simulink model "emrax208"  (R2024a)
settings: Solver=ode5  StartTime=0.0  StopTime=sim.time  FixedStep=sim.Ts  RelTol=1e-3
undefined symbols (not defined in the file or in its folder): c, ki, kp, sim, T_ref
libraries: slpidlib x2, simulink x1
settings Model: SimulationMode=accelerator  Creator=skh88  LastModifiedBy=skh88
settings SimscapeCC: ExplicitSolverDiagnosticOptions=none

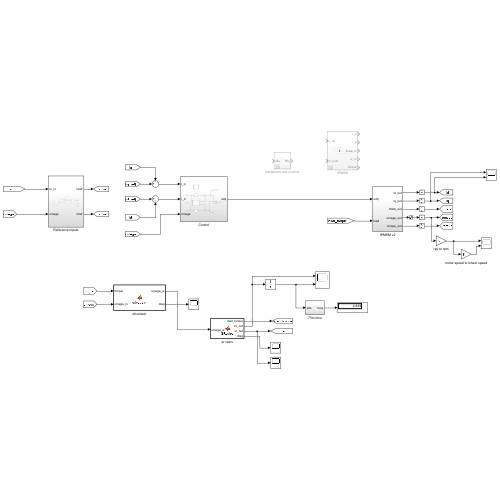
[thumbnail: Simulink's stored preview of the top-level diagram]
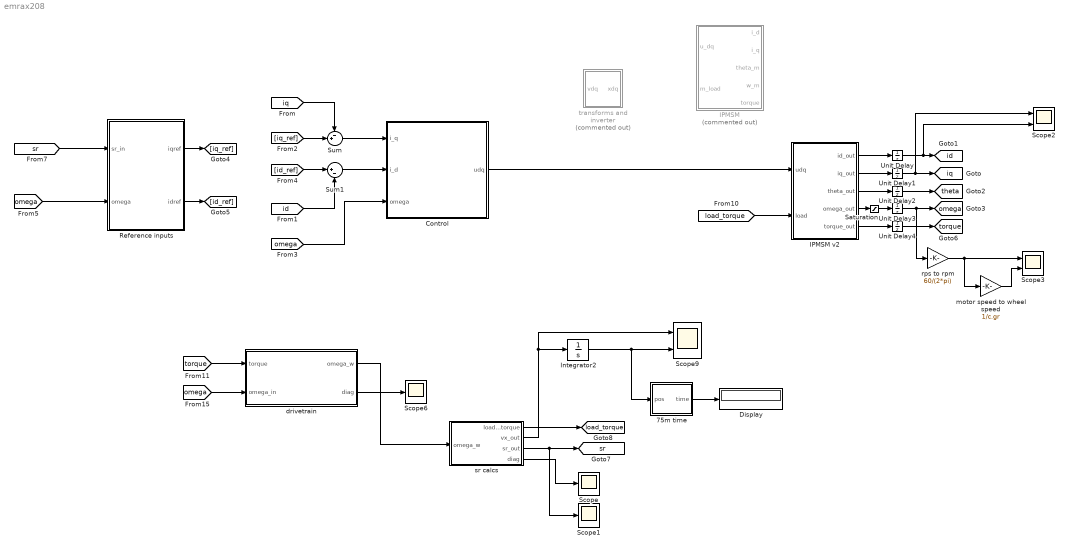
== system emrax208 ==
  75m time : Subsystem
  Control : Subsystem
  Display : Display
  IPMSM : Subsystem  Commented=on
  IPMSM v2 : Subsystem
  Integrator2 : Integrator
  Reference inputs : Subsystem
  Saturation : Saturate  UpperLimit=c.max_rpm  LowerLimit=0
  Scope : Scope
  Scope1 : Scope
  Scope2 : Scope  NumInputPorts=2
  Scope3 : Scope  NumInputPorts=2
  Scope6 : Scope
  Scope9 : Scope  NumInputPorts=2
  Sum : Sum  Inputs=-+|
  Sum1 : Sum  Inputs=|+-
  Unit Delay{,1..4} (5 alike) : UnitDelay  SampleTime=-1  HasFrameUpgradeWarning=on
  drivetrain : MATLAB Function  TreatAsAtomicUnit=on
  motor speed to wheel speed : Gain  Gain=1/c.gr
  rps to rpm : Gain  Gain=60/(2*pi)
  sr calcs : MATLAB Function  TreatAsAtomicUnit=on
  transforms and inverter : Subsystem  Commented=on
  tag scope: id=global, iq=global, load_torque=global, omega=global, sr=global, theta=global, torque=global
  wires:
  [iq] -> Sum/1
  [id] -> Sum1/2
  Reference inputs/1(iqref) -> [iq_ref]
  Reference inputs/2(idref) -> [id_ref]
  [iq_ref] -> Sum/2
  [id_ref] -> Sum1/1
  rps to rpm/1 -> Scope3/1, motor speed to wheel speed/1
  motor speed to wheel speed/1 -> Scope3/2
  Sum/1 -> Control/1(i_q)
  Sum1/1 -> Control/2(i_d)
  [omega] -> Control/3(omega)
  Unit Delay/1 -> Scope2/2, [id]
  Unit Delay1/1 -> Scope2/1, [iq]
  Unit Delay4/1 -> [torque]
  Unit Delay2/1 -> [theta]
  Unit Delay3/1 -> [omega], rps to rpm/1
  IPMSM v2/3(theta_out) -> Unit Delay2/1
  IPMSM v2/2(iq_out) -> Unit Delay1/1
  IPMSM v2/1(id_out) -> Unit Delay/1
  IPMSM v2/4(omega_out) -> Saturation/1
  IPMSM v2/5(torque_out) -> Unit Delay4/1
  Saturation/1 -> Unit Delay3/1
  [load_torque] -> IPMSM v2/2(load)
  sr calcs/2(vx_out) -> Integrator2/1, Scope9/1
  drivetrain/2(diag) -> Scope6/1
  Integrator2/1 -> 75m time/1(pos), Scope9/2
  sr calcs/4(diag) -> Scope/1
  drivetrain/1(omega_w) -> sr calcs/1(omega_w)
  75m time/1(time) -> Display/1
  [omega] -> drivetrain/2(omega_in)
  sr calcs/1(load_torque) -> [load_torque]
  sr calcs/3(sr_out) -> Scope1/1, [sr]
  [torque] -> drivetrain/1(torque)
  [sr] -> Reference inputs/1(sr_in)
  [omega] -> Reference inputs/2(omega)
  Control/1(udq) -> IPMSM v2/1(udq)

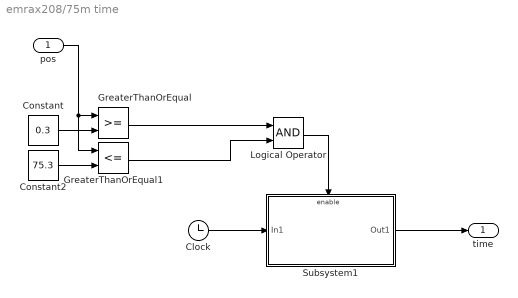
== system emrax208/75m time ==
  pos : Inport
  Clock : Clock
  Constant : Constant  Value=0.3
  Constant2 : Constant  Value=75.3
  GreaterThanOrEqual : RelationalOperator  OutDataTypeStr=boolean  RndMeth=Simplest  InputSameDT=off
  GreaterThanOrEqual1 : RelationalOperator  Operator=<=  OutDataTypeStr=boolean  RndMeth=Simplest  InputSameDT=off
  Logical Operator : Logic  AllPortsSameDT=off  OutDataTypeStr=boolean
  Subsystem1 : Subsystem
  time : Outport
  wires:
  Constant/1 -> GreaterThanOrEqual/2
  Logical Operator/1 -> Subsystem1/Enable
  GreaterThanOrEqual1/1 -> Logical Operator/2
  Clock/1 -> Subsystem1/1(In1)
  Constant2/1 -> GreaterThanOrEqual1/2
  Subsystem1/1(Out1) -> time/1
  GreaterThanOrEqual/1 -> Logical Operator/1
  pos/1 -> GreaterThanOrEqual1/1, GreaterThanOrEqual/1

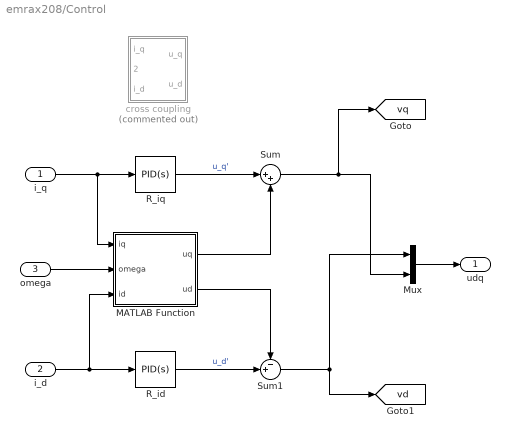
== system emrax208/Control ==
  i_q : Inport
  i_d : Inport  Port=2
  omega : Inport  Port=3
  MATLAB Function : MATLAB Function  TreatAsAtomicUnit=on
  Mux : Mux  Inputs=2
  R_id : slpidlib/PID Controller  Controller=PID  Form=Parallel  TimeDomain=Continuous-time  UseExternalTs=off  SampleTime=c.controllerTs  IntegratorMethod=Forward Euler  FilterMethod=Forward Euler  ControllerParametersSource=internal  P=kp  I=ki  UseKiTs=off  D=0  UseExternalDerivativeSource=off  N=100  UseFilter=on  TunerSelectOption=Transfer Function Based (PID Tuner App)  InitialConditionSource=internal  InitialConditionForIntegrator=0  InitialConditionForFilter=0  DifferentiatorICPrevScaledInput=0  ExternalReset=none  TrackingMode=off  Kt=1  LimitOutput=off  SatLimitsSource=internal  UpperSaturationLimit=2*c.R*c.I_nominal  LowerSaturationLimit=-2*c.R*c.I_nominal  LinearizeAsGain=on  AntiWindupMode=clamping  Kb=1  LimitIntegrator=off  UpperIntegratorSaturationLimit=2*c.R*c.I_nominal  LowerIntegratorSaturationLimit=-2*c.R*c.I_nominal  POutMin=[]  POutMax=[]  IOutMin=[]  IOutMax=[]  DOutMin=[]  DOutMax=[]  NOutMin=[]  NOutMax=[]  SumOutMin=[]  SumOutMax=[]  SaturationOutMin=[]  SaturationOutMax=[]  PParamMin=[]  PParamMax=[]  IParamMin=[]  IParamMax=[]  DParamMin=[]  DParamMax=[]  NParamMin=[]  NParamMax=[]  KbParamMin=[]  KbParamMax=[]  KtParamMin=[]  KtParamMax=[]  KbOutMin=[]  KbOutMax=[]  KtOutMin=[]  KtOutMax=[]  IntegratorOutMin=[]  IntegratorOutMax=[]  FilterOutMin=[]  FilterOutMax=[]  SumI1OutMin=[]  SumI1OutMax=[]  SumI2OutMin=[]  SumI2OutMax=[]  SumI3OutMin=[]  SumI3OutMax=[]  SumI4OutMin=[]  SumI4OutMax=[]  SumDOutMin=[]  SumDOutMax=[]  DifferentiatorOutMin=[]  DifferentiatorOutMax=[]  FilterDiffOutCoefMin=[]  FilterDiffOutCoefMax=[]  ReciprocalOutMin=[]  ReciprocalOutMax=[]  SumDenOutMin=[]  SumDenOutMax=[]  SumNumOutMin=[]  SumNumOutMax=[]  DivideOutMin=[]  DivideOutMax=[]  UdiffTsProdOutMin=[]  UdiffTsProdOutMax=[]  NTsProdOutMin=[]  NTsProdOutMax=[]  UintegralTsProdOutMin=[]  UintegralTsProdOutMax=[]  UngainTsProdOutMin=[]  UngainTsProdOutMax=[]  ClampingZeroOutDataTypeStr=Inherit: Inherit via back propagation  ClampingZeroOutMin=[]  ClampingZeroOutMax=[]  FilterDenConstantOutDataTypeStr=Inherit: Inherit via back propagation  FilterDenConstantOutMin=[]  FilterDenConstantOutMax=[]  PCopyOutDataTypeStr=Inherit: Inherit via back propagation  PCopyOutMin=[]  PCopyOutMax=[]  NCopyOutDataTypeStr=Inherit: Inherit via back propagation  NCopyOutMin=[]  NCopyOutMax=[]  IntegratorContinuousStateAttributes=''  IntegratorStateMustResolveToSignalObject=off  IntegratorRTWStateStorageClass=Auto  FilterContinuousStateAttributes=''  FilterStateMustResolveToSignalObject=off  FilterRTWStateStorageClass=Auto  ParallelPVariant=InternalParameters  IdealPVariant=Disabled  IVariant=InternalParameters  DVariant=InternalParameters  IntegratorVariant=Continuous  SatVariant=Disabled  AWVariant=Passthrough  PCopyVariant=Disabled  TRVariant=Disabled  FdbkBlocksVariant=Forward  IdealPFdbkVariant=Disabled  SatFdbkVariant=Disabled  DerivativeFilterVariant=ContFilter  NVariant=InternalParameters  NCopyVariant=Disabled  FilterICVariant=InternalICsFilter  IntegratorICVariant=InternalICs  ExternalResetVariant=Disabled  TRSumVariant=Passthrough  SumFdbkVariant=Disabled  SumVariant=Sum_PID  TsampFilterVariant=InternalTs  TsampNgainVariant=Passthrough  TsampIntegralVariant=Disabled_SignalSpec  ExternalSaturationOutDataTypeStr=Inherit: Same as second input  DerivativeSourceVariant=ErrorSignal
  R_iq : slpidlib/PID Controller  Controller=PID  Form=Parallel  TimeDomain=Continuous-time  UseExternalTs=off  SampleTime=c.controllerTs  IntegratorMethod=Forward Euler  FilterMethod=Forward Euler  ControllerParametersSource=internal  P=kp  I=ki  UseKiTs=off  D=0  UseExternalDerivativeSource=off  N=100  UseFilter=on  TunerSelectOption=Transfer Function Based (PID Tuner App)  InitialConditionSource=internal  InitialConditionForIntegrator=0  InitialConditionForFilter=0  DifferentiatorICPrevScaledInput=0  ExternalReset=none  TrackingMode=off  Kt=1  LimitOutput=off  SatLimitsSource=internal  UpperSaturationLimit=c.max_rpm*c.p*c.lambda  LowerSaturationLimit=-c.max_rpm*c.p*c.lambda  LinearizeAsGain=on  AntiWindupMode=clamping  Kb=1  LimitIntegrator=off  UpperIntegratorSaturationLimit=c.max_rpm*c.p*c.lambda  LowerIntegratorSaturationLimit=-c.max_rpm*c.p*c.lambda  POutMin=[]  POutMax=[]  IOutMin=[]  IOutMax=[]  DOutMin=[]  DOutMax=[]  NOutMin=[]  NOutMax=[]  SumOutMin=[]  SumOutMax=[]  SaturationOutMin=[]  SaturationOutMax=[]  PParamMin=[]  PParamMax=[]  IParamMin=[]  IParamMax=[]  DParamMin=[]  DParamMax=[]  NParamMin=[]  NParamMax=[]  KbParamMin=[]  KbParamMax=[]  KtParamMin=[]  KtParamMax=[]  KbOutMin=[]  KbOutMax=[]  KtOutMin=[]  KtOutMax=[]  IntegratorOutMin=[]  IntegratorOutMax=[]  FilterOutMin=[]  FilterOutMax=[]  SumI1OutMin=[]  SumI1OutMax=[]  SumI2OutMin=[]  SumI2OutMax=[]  SumI3OutMin=[]  SumI3OutMax=[]  SumI4OutMin=[]  SumI4OutMax=[]  SumDOutMin=[]  SumDOutMax=[]  DifferentiatorOutMin=[]  DifferentiatorOutMax=[]  FilterDiffOutCoefMin=[]  FilterDiffOutCoefMax=[]  ReciprocalOutMin=[]  ReciprocalOutMax=[]  SumDenOutMin=[]  SumDenOutMax=[]  SumNumOutMin=[]  SumNumOutMax=[]  DivideOutMin=[]  DivideOutMax=[]  UdiffTsProdOutMin=[]  UdiffTsProdOutMax=[]  NTsProdOutMin=[]  NTsProdOutMax=[]  UintegralTsProdOutMin=[]  UintegralTsProdOutMax=[]  UngainTsProdOutMin=[]  UngainTsProdOutMax=[]  ClampingZeroOutDataTypeStr=Inherit: Inherit via back propagation  ClampingZeroOutMin=[]  ClampingZeroOutMax=[]  FilterDenConstantOutDataTypeStr=Inherit: Inherit via back propagation  FilterDenConstantOutMin=[]  FilterDenConstantOutMax=[]  PCopyOutDataTypeStr=Inherit: Inherit via back propagation  PCopyOutMin=[]  PCopyOutMax=[]  NCopyOutDataTypeStr=Inherit: Inherit via back propagation  NCopyOutMin=[]  NCopyOutMax=[]  IntegratorContinuousStateAttributes=''  IntegratorStateMustResolveToSignalObject=off  IntegratorRTWStateStorageClass=Auto  FilterContinuousStateAttributes=''  FilterStateMustResolveToSignalObject=off  FilterRTWStateStorageClass=Auto  ParallelPVariant=InternalParameters  IdealPVariant=Disabled  IVariant=InternalParameters  DVariant=InternalParameters  IntegratorVariant=Continuous  SatVariant=Disabled  AWVariant=Passthrough  PCopyVariant=Disabled  TRVariant=Disabled  FdbkBlocksVariant=Forward  IdealPFdbkVariant=Disabled  SatFdbkVariant=Disabled  DerivativeFilterVariant=ContFilter  NVariant=InternalParameters  NCopyVariant=Disabled  FilterICVariant=InternalICsFilter  IntegratorICVariant=InternalICs  ExternalResetVariant=Disabled  TRSumVariant=Passthrough  SumFdbkVariant=Disabled  SumVariant=Sum_PID  TsampFilterVariant=InternalTs  TsampNgainVariant=Passthrough  TsampIntegralVariant=Disabled_SignalSpec  ExternalSaturationOutDataTypeStr=Inherit: Same as second input  DerivativeSourceVariant=ErrorSignal
  Sum : Sum  Inputs=|++
  Sum1 : Sum  Inputs=-+|
  cross coupling : Subsystem  Commented=on
  udq : Outport
  tag scope: vd=global, vq=global
  wires:
  R_id/1 -> Sum1/2  "u_d'"
  R_iq/1 -> Sum/1  "u_q'"
  i_d/1 -> MATLAB Function/3(id), R_id/1
  i_q/1 -> MATLAB Function/1(iq), R_iq/1
  Sum/1 -> [vq], Mux/2
  omega/1 -> MATLAB Function/2(omega)
  MATLAB Function/1(uq) -> Sum/2
  MATLAB Function/2(ud) -> Sum1/1
  Sum1/1 -> [vd], Mux/1
  Mux/1 -> udq/1

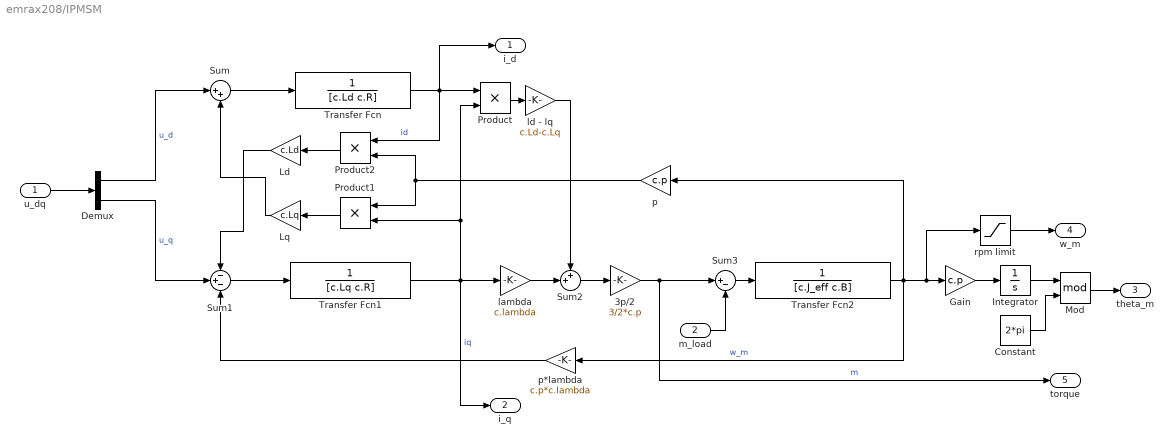
== system emrax208/IPMSM ==
  u_dq : Inport
  m_load : Inport  Port=2
  3p/2 : Gain  Gain=3/2*c.p
  Constant : Constant  Value=2*pi
  Demux : Demux  Outputs=2
  Gain : Gain  Gain=c.p
  Integrator : Integrator
  Ld : Gain  Gain=c.Ld
  Lq : Gain  Gain=c.Lq
  Mod : Math  Operator=mod
  Product : Product
  Product1 : Product
  Product2 : Product
  Sum : Sum  Inputs=|++
  Sum1 : Sum  Inputs=-+-
  Sum2 : Sum  Inputs=++|
  Sum3 : Sum  Inputs=|+-
  Transfer Fcn : TransferFcn  Denominator=[c.Ld c.R]
  Transfer Fcn1 : TransferFcn  Denominator=[c.Lq c.R]
  Transfer Fcn2 : TransferFcn  Denominator=[c.J_eff c.B]
  lambda : Gain  Gain=c.lambda
  ld - lq : Gain  Gain=c.Ld-c.Lq
  p : Gain  Gain=c.p
  p*lambda : Gain  Gain=c.p*c.lambda
  rpm limit : Saturate  UpperLimit=c.max_rpm  LowerLimit=0
  i_d : Outport
  i_q : Outport  Port=2
  theta_m : Outport  Port=3
  w_m : Outport  Port=4
  torque : Outport  Port=5
  wires:
  m_load/1 -> Sum3/2
  Transfer Fcn1/1 -> Product1/2, Product/2, lambda/1, i_q/1  "iq"
  Product2/1 -> Ld/1
  Transfer Fcn/1 -> Product2/1, Product/1, i_d/1  "id"
  p/1 -> Product1/1, Product2/2
  Sum1/1 -> Transfer Fcn1/1
  Sum/1 -> Transfer Fcn/1
  3p/2/1 -> torque/1, Sum3/1  "m"
  Sum3/1 -> Transfer Fcn2/1
  Transfer Fcn2/1 -> p*lambda/1, p/1, Gain/1, rpm limit/1  "w_m"
  lambda/1 -> Sum2/2
  Product1/1 -> Lq/1
  Lq/1 -> Sum/2
  Ld/1 -> Sum1/1
  p*lambda/1 -> Sum1/3
  Integrator/1 -> Mod/1
  rpm limit/1 -> w_m/1
  Demux/1 -> Sum/1  "u_d"
  Demux/2 -> Sum1/2  "u_q"
  u_dq/1 -> Demux/1
  Gain/1 -> Integrator/1
  ld - lq/1 -> Sum2/1
  Sum2/1 -> 3p/2/1
  Product/1 -> ld - lq/1
  Constant/1 -> Mod/2
  Mod/1 -> theta_m/1

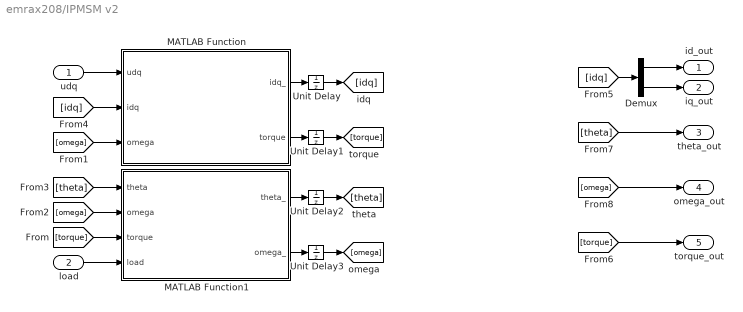
== system emrax208/IPMSM v2 ==
  udq : Inport
  load : Inport  Port=2
  Demux : Demux  Outputs=2
  MATLAB Function : MATLAB Function  TreatAsAtomicUnit=on
  MATLAB Function1 : MATLAB Function  TreatAsAtomicUnit=on
  Unit Delay{,1..3} (4 alike) : UnitDelay  SampleTime=-1  HasFrameUpgradeWarning=on
  id_out : Outport
  iq_out : Outport  Port=2
  theta_out : Outport  Port=3
  omega_out : Outport  Port=4
  torque_out : Outport  Port=5
  wires:
  MATLAB Function/2(torque) -> Unit Delay1/1
  [torque] -> MATLAB Function1/3(torque)
  MATLAB Function1/2(omega_) -> Unit Delay3/1
  [omega] -> MATLAB Function/3(omega)
  [omega] -> MATLAB Function1/2(omega)
  MATLAB Function1/1(theta_) -> Unit Delay2/1
  [theta] -> MATLAB Function1/1(theta)
  load/1 -> MATLAB Function1/4(load)
  udq/1 -> MATLAB Function/1(udq)
  MATLAB Function/1(idq_) -> Unit Delay/1
  [idq] -> MATLAB Function/2(idq)
  [idq] -> Demux/1
  [torque] -> torque_out/1
  [theta] -> theta_out/1
  Demux/1 -> id_out/1
  Demux/2 -> iq_out/1
  Unit Delay/1 -> [idq]
  Unit Delay1/1 -> [torque]
  Unit Delay2/1 -> [theta]
  [omega] -> omega_out/1
  Unit Delay3/1 -> [omega]

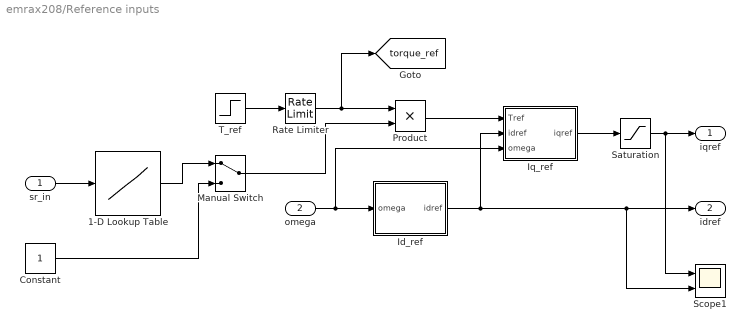
== system emrax208/Reference inputs ==
  sr_in : Inport
  omega : Inport  Port=2
  1-D Lookup Table : Lookup_n-D  NumberOfTableDimensions=1  BreakpointsForDimension1=linspace(0, 0.5, 100)  Table=(-tanh(linspace(-3, 3, 100))+1)/2  InternalRulePriority=Speed  RndMeth=Simplest
  Constant : Constant
  Id_ref : MATLAB Function  TreatAsAtomicUnit=on
  Iq_ref : MATLAB Function  TreatAsAtomicUnit=on
  Manual Switch : ManualSwitch
  Product : Product
  Rate Limiter : RateLimiter  RisingSlewLimit=5e3  FallingSlewLimit=-5e3  SampleTimeMode=inherited
  Saturation : Saturate  UpperLimit=c.I_peak  LowerLimit=-c.I_peak
  Scope1 : Scope  NumInputPorts=2
  T_ref : Step  Time=0  After=T_ref  SampleTime=sim.Ts
  iqref : Outport
  idref : Outport  Port=2
  tag scope: torque_ref=global
  wires:
  Id_ref/1(idref) -> Scope1/2, idref/1, Iq_ref/2(idref)
  Iq_ref/1(iqref) -> Saturation/1
  Saturation/1 -> Scope1/1, iqref/1
  T_ref/1 -> Rate Limiter/1
  Rate Limiter/1 -> [torque_ref], Product/1
  sr_in/1 -> 1-D Lookup Table/1
  Product/1 -> Iq_ref/1(Tref)
  1-D Lookup Table/1 -> Manual Switch/1
  Constant/1 -> Manual Switch/2
  omega/1 -> Iq_ref/3(omega), Id_ref/1(omega)
  Manual Switch/1 -> Product/2

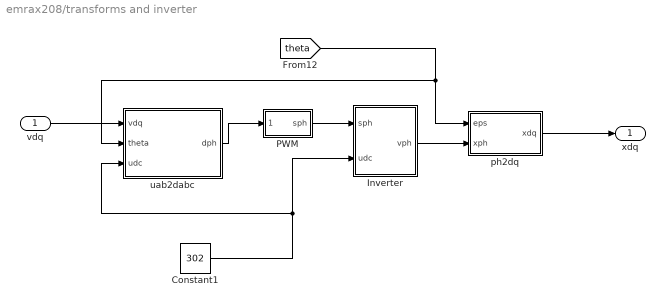
== system emrax208/transforms and inverter ==
  vdq : Inport
  Constant1 : Constant  Value=302  SampleTime=Inf
  Inverter : MATLAB Function  TreatAsAtomicUnit=on
  PWM : Subsystem
  ph2dq : MATLAB Function  TreatAsAtomicUnit=on
  uab2dabc : MATLAB Function  TreatAsAtomicUnit=on
  xdq : Outport
  wires:
  Constant1/1 -> Inverter/2(udc), uab2dabc/3(udc)
  [theta] -> ph2dq/1(eps), uab2dabc/2(theta)
  ph2dq/1(xdq) -> xdq/1
  Inverter/1(vph) -> ph2dq/2(xph)
  uab2dabc/1(dph) -> PWM/1(dph)
  PWM/1(sph) -> Inverter/1(sph)
  vdq/1 -> uab2dabc/1(vdq)

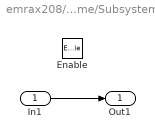
== system emrax208/75m time/Subsystem1 ==
  In1 : Inport
  Enable : EnablePort
  Out1 : Outport
  wires:
  In1/1 -> Out1/1

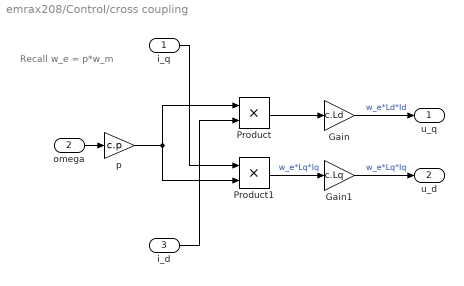
== system emrax208/Control/cross coupling ==
  note: Recall w_e = p*w_m
  i_q : Inport
  omega : Inport  Port=2
  i_d : Inport  Port=3
  Gain : Gain  Gain=c.Ld
  Gain1 : Gain  Gain=c.Lq
  Product : Product
  Product1 : Product
  p : Gain  Gain=c.p
  u_q : Outport
  u_d : Outport  Port=2
  wires:
  i_d/1 -> Product/2
  omega/1 -> p/1
  Gain/1 -> u_q/1  "w_e*Ld*Id"
  i_q/1 -> Product1/1
  Gain1/1 -> u_d/1  "w_e*Lq*Iq"
  p/1 -> Product/1, Product1/2
  Product/1 -> Gain/1
  Product1/1 -> Gain1/1  "w_e*Lq*Iq"

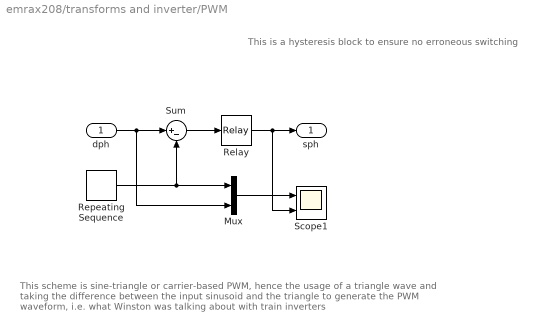
== system emrax208/transforms and inverter/PWM ==
  note: This scheme is sine-triangle or carrier-based PWM, hence the usage of a triangle wave and taking the difference between the input sinusoid and the triangle to generate the PWM waveform, i.e. what Winston was talking about with train inverters
  note: This is a hysteresis block to ensure no erroneous switching
  dph : Inport
  Mux : Mux  Inputs=2
  Relay : Relay  OnSwitchValue=2e-10  OffSwitchValue=-2e-10
  Repeating Sequence : simulink/Sources/Repeating Sequence  rep_seq_t=[0 c.Ts/2 c.Ts]  rep_seq_y=[0 1 0]
  Scope1 : Scope  NumInputPorts=2
  Sum : Sum  Inputs=|+-
  sph : Outport
  wires:
  Sum/1 -> Relay/1
  Repeating Sequence/1 -> Mux/1, Sum/2
  dph/1 -> Mux/2, Sum/1
  Relay/1 -> sph/1, Scope1/2
  Mux/1 -> Scope1/1

== matlab function emrax208/Reference inputs/Id_ref ==
  data: omega input; idref output; c parameter
function idref = fcn(omega, c)

idref = 0;

if omega*c.p >= c.omega_base
    idref = (c.omega_base-omega*c.p)*c.lambda/(omega*c.p*c.Ld);
    idref = max(idref, -c.I_lim);
end

== matlab function emrax208/transforms and inverter/ph2dq ==
  data: eps input; xdq output size=[2,1]; xph input
function xdq  = ph2dq(eps,xph)
  % Synchronous reference frame transformation  
  
  % Space Vector Transformation (Clarke)
  xab=[0;0];
  xab(1)= 2/3*xph(1) - 1/3*(xph(2)+xph(3)); 
  xab(2)= 1/sqrt(3)* (xph(2)-xph(3));
  
  % Direct Vector Calculation (Park)
  xdq=[0;0];
  xdq(1)=  xab(1)*cos(eps) + xab(2)*sin(eps);
  xdq(2)= -xab(1)*sin(eps) + xab(2)*cos(eps);

== matlab function emrax208/IPMSM v2/MATLAB Function ==
  data: idq_ output size=2; torque output size=1; udq input; idq input; omega input; c parameter
function [idq_, torque] = ipmsm_electrical(udq, idq, omega, c)

vd = udq(1) - c.R*idq(1);
vq = udq(2) - c.R*idq(2);

id = (c.Tstep*vd + c.Ld*idq(1) + c.Tstep*omega*c.p*c.Lq*idq(2))/c.Ld;
iq = (c.Tstep*vq + c.Lq*idq(2) - c.Tstep*omega*c.p*(c.Ld*idq(1) + c.lambda))/c.Lq;

idq_ = [id;iq];

torque = 3/2*c.p*(c.lambda*iq + (c.Ld - c.Lq)*id*iq);

== matlab function emrax208/transforms and inverter/uab2dabc ==
  data: dph output size=3; vdq input; theta input; udc input
function dph = fcn(vdq,theta,udc)
%#codegen

% Inverse Park
vab = zeros(2,1);
vab(1) = cos(theta)*vdq(1) -sin(theta)*vdq(2);
vab(2) = sin(theta)*vdq(1) +cos(theta)*vdq(2);

% Inverse Clarke
vph = zeros(3,1);
vph(1) = vab(1);
vph(2) = -1/2*vab(1) +sqrt(3)/2*vab(2);
vph(3) = -1/2*vab(1) -sqrt(3)/2*vab(2);

% modulation index
mph = vph/(udc/2);
% duty cycle
dph = (mph+1)/2;

% limitation
for i=1:3
    if dph(i) > 1
        dph(i) = 1;
    elseif dph(i) < 0
        dph(i) = 0;
    end
end

% backcalculation of applied voltage
vphsat = (2*dph-1)*udc/2;  % m=(2*dph-1)

vabsat = zeros(2,1);
vabsat(1) = 2/3*vphsat(1) -1/3*vphsat(2) -1/3*vphsat(3);
vabsat(2) = 1/sqrt(3)*vphsat(2) -1/sqrt(3)*vphsat(3);

vdqsat = zeros(2,1);
vdqsat(1) =  cos(theta)*vabsat(1) +sin(theta)*vabsat(2);
vdqsat(2) = -sin(theta)*vabsat(1) +cos(theta)*vabsat(2);

== matlab function emrax208/transforms and inverter/Inverter ==
  data: sph input; vph output; udc input
function vph  = fcn(sph,udc)
%#codegen

vph = (2*sph-1)*udc/2;

== matlab function emrax208/IPMSM v2/MATLAB Function1 ==
  data: theta_ output; omega_ output; theta input; omega input; torque input; load input; c parameter
function [theta_, omega_] = ipmsm_mechanical(theta, omega, torque, load, c)

omega_ = c.Tstep/c.J*(torque - load - c.B*omega) + omega;
theta_ = mod(theta + c.Tstep*c.p*omega, 2*pi);

== matlab function emrax208/Reference inputs/Iq_ref ==
  data: Tref input; idref input; omega input; iqref output; c parameter
function iqref = fcn(Tref, idref, omega, c)
% Current reference generation using the torque equation
% Inputs:
%  - Tref: torque reference
%  - idref: d-current reference
% Output
%  - iqref

% Using torque equation for IPMSM
iqref = 2*Tref/(3*c.p*(c.lambda + (c.Ld - c.Lq)*idref));

if omega*c.p >= c.omega_base
    iqref = min(iqref, sqrt(c.I_lim^2-idref^2));
end

== matlab function emrax208/Control/MATLAB Function ==
  data: uq output; iq input; omega input; id input; ud output; c parameter
function [uq, ud] = crosscouple(iq, omega, id, c)

ud = c.Lq*c.p*omega*iq;
uq = c.Ld*c.p*omega*id;

== matlab function emrax208/drivetrain ==
  data: torque input; omega_in input; omega_w output; c parameter; diag output
function [omega_w, diag] = drivetrain(torque, omega_in, c)

g = 9.81;

persistent omega_prev;
if isempty(omega_prev)
    omega_prev = 0;
end

% Predict motor omega
omega_dynamical = c.Tstep/(c.J_eff)*(c.eta*torque - c.B*omega_prev) + omega_prev;
omega_pred = omega_prev + (omega_dynamical - omega_prev)*c.Tstep;

% Estimate motor omega
omega_weight = 0.5;
omega_ = omega_weight*omega_pred + (1-omega_weight)*omega_in;

omega_prev = omega_;
omega_w = omega_/c.gr;

% DIAGNOSTIC OUTPUT TO SCOPE
diag = omega_w*60/(2*pi);

== matlab function emrax208/sr calcs ==
  data: load_torque output; vx_out output; sr_out output; omega_w input; c parameter; diag output
function [load_torque, vx_out, sr_out, diag] = SRcalcs(omega_w, c)

% Constants
g = 9.81;
dt = c.Tstep;
f_static = c.m*g*c.distrib;
mu = 1.22;
B = c.bx; C = c.cx; D = c.dx; E = c.ex;
% scale1 = 1-(omega_w*c.gr/c.max_rpm);
% scale2 = torque/140;

persistent sr vx ax f_tract;

if isempty(ax)
    ax = mu*g*c.distrib;
end

if isempty(f_tract)
    f_tract = 0;
end

if isempty(vx)
    vx = 0;
end

if isempty(sr)
    sr = 0;
end

lt = c.m*ax*c.cg/c.wb;
f_norm = f_static + lt;
f_tract1 = mu*f_norm;

axtemp = f_tract1/c.m;
vxtemp = vx + axtemp*dt;

if vxtemp ~= 0 && omega_w > 0
    srtemp = max((omega_w*c.r - vxtemp)/vxtemp, 0);
else
    srtemp = 0;
end

% Recalculate using pacejka
fx_pacejka = D*sin(C*atan(B*srtemp - E*(B*srtemp - atan(B*srtemp)))); % absolute max tractive force of one wheel
fx_pacejka = fx_pacejka*2*2/3; % scale for sandpaper belt, mult by 2 for total tractive force

% Okay suddenly we don't need this???
% f_tract2 = fx_pacejka;
% weight = 1-scale1;
% f_tract = weight*f_tract1 + (1-weight)*f_tract2; % weight both tractive force calcs

f_tract = fx_pacejka;
ax = f_tract/c.m;
vx = vx + ax*dt;

if vx ~= 0 && omega_w > 0
    sr = max((omega_w*c.r - vx)/vx, 0);
end

vx_out = vx;
load_torque = f_tract*c.r/(c.eta*c.gr);

sr_out = sr;

diag = ax/g;
